simulink model "SFS"  (R2026a)
settings: Solver=ode23t  StopTime=pp.t_stop  AbsTol=1e-3
PreLoadFcn:
  | addpath(fileparts(which('SFS')));
  | pp = protectionParams();
InitFcn:
  | addpath(fileparts(which('SFS')));
  | pp = protectionParams();
undefined symbols (not defined in the file or in its folder): DiscIntNeverNeededParam
libraries: ee_lib x5, fl_lib x4, nesl_utility x4
settings Model: Creator=smred  LastModifiedBy=smred
settings DebuggingCC: SymbolicDimsDataTypeCodeGenerationDiagnostic=none
settings SimscapeCC: SimscapeLogDecimation=50.0

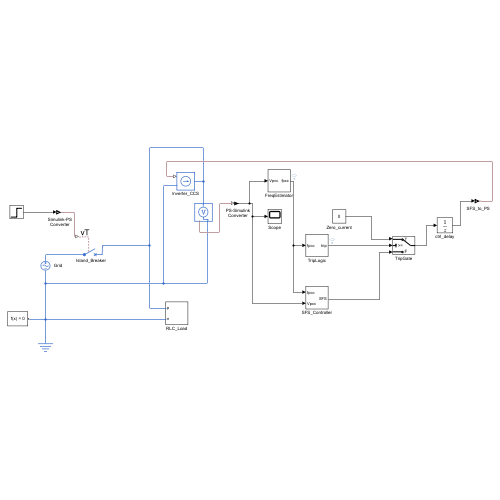
[thumbnail: Simulink's stored preview of the top-level diagram]
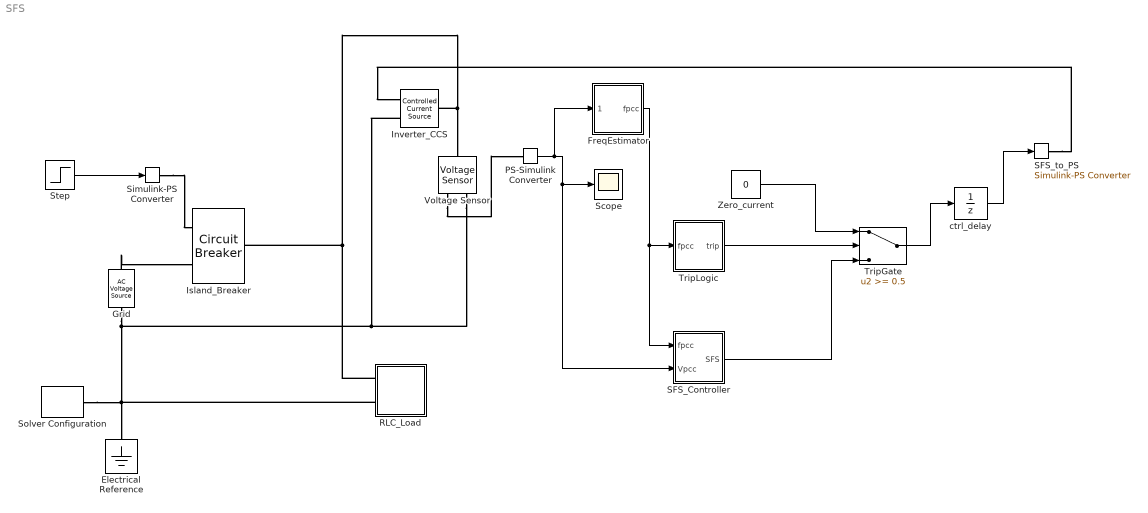
== system SFS ==
  Electrical Reference : fl_lib/Electrical/Electrical Elements/Electrical Reference
  FreqEstimator : Subsystem
  Grid : fl_lib/Electrical/Electrical Sources/AC Voltage Source  amp=pp.Vg_amp V  shift=0 deg  frequency=pp.f_n Hz
  Inverter_CCS : fl_lib/Electrical/Electrical Sources/Controlled Current Source
  Island_Breaker : ee_lib/Switches & Breakers/Circuit Breaker  R_closed=0.001 Ohm  G_open=1e-6 1/Ohm  threshold=0.5 V  breaker_behavior=ee.enum.switches.breakerBehavior.zeroCrossingDisable  port_option=ee.enum.threePhasePort.composite  control_port_option=ee.enum.controlport.ps  i_th=1e-8 A
  PS-Simulink Converter : nesl_utility/PS-Simulink Converter  PhysicalDomain=network_engine_domain  SubClassName=ps_output  LeftPortType=input  RightPortType=output  PseudoPeriodic=off  Frequencies=[]  VectorFormat=inherit  Unit=inherit  AffineConversion=off
  RLC_Load : Subsystem
  SFS_Controller : Subsystem
  SFS_to_PS : nesl_utility/Simulink-PS Converter  PhysicalDomain=network_engine_domain  SubClassName=ps_input  LeftPortType=input  RightPortType=output  PseudoPeriodic=off  Frequencies=[]  NoiseDistribution=none  NoiseParameters=[]  Unit=1  AffineConversion=off  FilteringAndDerivatives=zero  SimscapeFilterOrder=1  InputFilterTimeConstant=0.001  UdotUserProvided=0
  Scope : Scope
      settings: ActiveDisplayYMinimum=-408.578503188974  ActiveDisplayYMaximum=411.2206775988297
  Simulink-PS Converter : nesl_utility/Simulink-PS Converter  PhysicalDomain=network_engine_domain  SubClassName=ps_input  LeftPortType=input  RightPortType=output  PseudoPeriodic=off  Frequencies=[]  NoiseDistribution=none  NoiseParameters=[]  Unit=1  AffineConversion=off  FilteringAndDerivatives=provide  SimscapeFilterOrder=1  InputFilterTimeConstant=0.001  UdotUserProvided=0
  Solver Configuration : nesl_utility/Solver Configuration  PhysicalDomain=network_engine_domain  SubClassName=solver  LeftPortType=input  RightPortType=generic  Tones=[]  Harmonics=[]  SimulateNoise=off  Profile=off  UseLocalSampling=off  EnableSwitchedLinearOptims=on  FrequencyDomain=off  UseCCode=off  RelTol=0.001  AbsTol=0.001  MinStep=1e-09  ToWorkspace=off  RevertToSquareIcSolve=off  NumHomotopyIterations=100  PhasorMode=off  PhasorModeNumHarmonics=1  ConsistencySolver=NEWTON_XTOL_AFTER_FTOL  CanonicalOrdering=CANONICAL  OptimizeIntermediates=OPTIMIZED  IndexReductionMethod=DerivativeReplacement  DoDC=off  ResidualTolerance=1e-09  ConsistencyTolSource=GLOBAL  ConsistencyAbsTol=0.001  ConsistencyRelTol=0.001  ConsistencyTolFactor=0.001  UseLocalSolver=off  LocalSolverChoice=NE_BACKWARD_EULER_ADVANCER  ResolveIndetEquations=on  FunctionEvalNumThread=1  LocalSolverSampleTime=0.001  DoFixedCost=off  MaxNonlinIter=3  MaxModeIter=2  ComputeImpulses=off  ImpulseIterations=2  LinearAlgebra=auto  LinearAlgebraNumThread=0  EquationFormulation=NE_TIME_EF  DelaysMemoryBudget=1024  AutomaticFiltering=on  FilteringTimeConstant=0.001  PartitionStorageMethod=AS_NEEDED  PartitionMemoryBudget=1024  PartitionMethod=ROBUST  MultibodyUseLocalSolver=off  MultibodyLocalSolverChoice=ODE1  MultibodyLocalSolverSampleTime=0.001
  Step : Step  Time=pp.t_island  SampleTime=0
  TripGate : Switch  Threshold=0.5  SaturateOnIntegerOverflow=off  InputSameDT=off
  TripLogic : Subsystem
  Voltage Sensor : fl_lib/Electrical/Electrical Sensors/Voltage Sensor
  Zero_current : Constant  Value=0
  ctrl_delay : UnitDelay  SampleTime=pp.Ts
  wires:
  Step/1 -> Simulink-PS Converter/1
  ctrl_delay/1 -> SFS_to_PS/1
  FreqEstimator/1(fpcc) -> SFS_Controller/1(fpcc), TripLogic/1(fpcc)
  SFS_Controller/1(SFS) -> TripGate/3
  PS-Simulink Converter/1 -> Scope/1, SFS_Controller/2(Vpcc), FreqEstimator/1(Vpcc)
  Zero_current/1 -> TripGate/1
  TripLogic/1(trip) -> TripGate/2
  TripGate/1 -> ctrl_delay/1
  connections:
  Voltage Sensor/RConn2 -- Inverter_CCS/RConn2 -- Electrical Reference/LConn1 -- Solver Configuration/RConn1 -- RLC_Load/LConn2 -- Grid/RConn1
  Grid/LConn1 -- Island_Breaker/LConn2
  Simulink-PS Converter/RConn1 -- Island_Breaker/LConn1
  Island_Breaker/RConn1 -- Inverter_CCS/LConn1 -- Voltage Sensor/LConn1 -- RLC_Load/LConn1
  Voltage Sensor/RConn1 -- PS-Simulink Converter/LConn1
  SFS_to_PS/RConn1 -- Inverter_CCS/RConn1

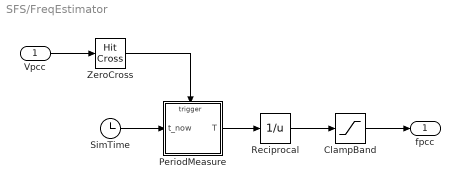
== system SFS/FreqEstimator ==
  Vpcc : Inport
  ClampBand : Saturate  UpperLimit=55  LowerLimit=45
  PeriodMeasure : Subsystem
  Reciprocal : Math  Operator=reciprocal
  SimTime : Clock
  ZeroCross : HitCross  HitCrossingDirection=rising
  fpcc : Outport
  wires:
  ClampBand/1 -> fpcc/1
  Reciprocal/1 -> ClampBand/1
  PeriodMeasure/1(T) -> Reciprocal/1
  ZeroCross/1 -> PeriodMeasure/Trigger
  SimTime/1 -> PeriodMeasure/1(t_now)
  Vpcc/1 -> ZeroCross/1

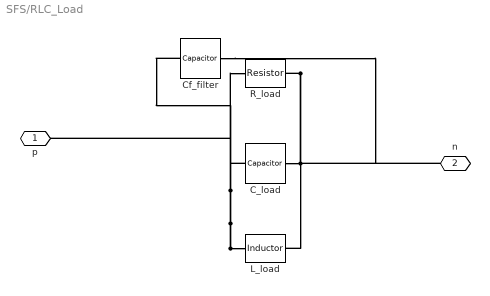
== system SFS/RLC_Load ==
  C_load : ee_lib/Passive/Capacitor  cap_option=ee.enum.passive.capacitor.capOption.const  c=pp.C_load F  Cvec=[1e-05, 1e-06] F  Vvec=[0, 10] V  CV_table_symmetry=ee.enum.passive.capacitor.tableSymmetry.yes  f_vec=[1, 10] kHz  DFext_vec=[.8, 1.2]  enable_C_tol=ee.enum.toleranceApplication.none  averaging_period=0 s  C_tol=5  tol_distribution=ee.enum.toleranceDistribution.uniform  nSigma=4  r=0 Ohm  g=0 1/Ohm  enable_operating_limits=ee.enum.enable.no  operating_limit_action=ee.enum.passive.reportOpLim.warn  max_working_voltage_range=[-25, 25] V  power_rating=1 W  maxTemperature=85 degC  thermalEnable=false  thermalMass=1 J/K  i_specify=off  i_priority=None  i=0 A  i_nominal_specify=off  i_nominal_value=1  i_nominal_unit=A  v_specify=off  v_priority=None  v=0 V  v_nominal_specify=off  v_nominal_value=1  v_nominal_unit=V  vc_specify=off  vc_priority=High  vc=0 V  vc_nominal_specify=off  vc_nominal_value=1  vc_nominal_unit=V  T_specify=off  T_priority=None  T=298.15 K  T_nominal_specify=off  T_nominal_value=1  T_nominal_unit=K
  Cf_filter : ee_lib/Passive/Capacitor  cap_option=ee.enum.passive.capacitor.capOption.const  c=pp.Cf F  Cvec=[1e-05, 1e-06] F  Vvec=[0, 10] V  CV_table_symmetry=ee.enum.passive.capacitor.tableSymmetry.yes  f_vec=[1, 10] kHz  DFext_vec=[.8, 1.2]  enable_C_tol=ee.enum.toleranceApplication.none  averaging_period=0 s  C_tol=5  tol_distribution=ee.enum.toleranceDistribution.uniform  nSigma=4  r=0 Ohm  g=0 1/Ohm  enable_operating_limits=ee.enum.enable.no  operating_limit_action=ee.enum.passive.reportOpLim.warn  max_working_voltage_range=[-25, 25] V  power_rating=1 W  maxTemperature=85 degC  thermalEnable=false  thermalMass=1 J/K  i_specify=off  i_priority=None  i=0 A  i_nominal_specify=off  i_nominal_value=1  i_nominal_unit=A  v_specify=off  v_priority=None  v=0 V  v_nominal_specify=off  v_nominal_value=1  v_nominal_unit=V  vc_specify=off  vc_priority=High  vc=0 V  vc_nominal_specify=off  vc_nominal_value=1  vc_nominal_unit=V  T_specify=off  T_priority=None  T=298.15 K  T_nominal_specify=off  T_nominal_value=1  T_nominal_unit=K
  L_load : ee_lib/Passive/Inductor  l=pp.L_load H  enable_L_tol=ee.enum.toleranceApplication.none  L_tol=20  tol_distribution=ee.enum.toleranceDistribution.uniform  nSigma=4  r=0 Ohm  g=1e-9 1/Ohm  enable_operating_limits=ee.enum.enable.no  operating_limit_action=ee.enum.passive.reportOpLim.warn  max_working_current=1 A  power_rating=1 W  i_L_specify=on  i_L_priority=High  i_L=pp.iL0 A  i_L_nominal_specify=off  i_L_nominal_value=1  i_L_nominal_unit=A
  R_load : ee_lib/Passive/Resistor  R=pp.R_load Ohm  enable_R_tol=ee.enum.toleranceApplication.none  R_tol=5  tol_distribution=ee.enum.toleranceDistribution.uniform  nSigma=4  enable_operating_limits=ee.enum.enable.no  operating_limit_action=ee.enum.passive.reportOpLim.warn  power_rating=1 W  max_working_voltage=100 V  noise_mode=ee.enum.sources.noise.Disabled  Tdevice=25 degC  sample_time=1e-3 s  repeatability=ee.enum.ic.repeatability.notRepeatable  user_seed=0  auto_seed=1045931777  power_derating_T1=70 degC  power_derating_T2=155 degC  operating_temperature_range_vec=[-50, 150] degC  alpha=3.93e-3 1/K  Tmeas=25 degC  thermal_mass=100 J/K  temperature_specify=off  temperature_priority=High  temperature=298.15 K  temperature_nominal_specify=off  temperature_nominal_value=1  temperature_nominal_unit=K
  p : PMIOPort  Side=Left
  n : PMIOPort  Port=2  Side=Left
  connections:
  L_load/LConn1 -- Cf_filter/LConn1 -- R_load/LConn1 -- p/RConn1 -- C_load/LConn1
  R_load/RConn1 -- n/RConn1 -- Cf_filter/RConn1 -- L_load/RConn1 -- C_load/RConn1

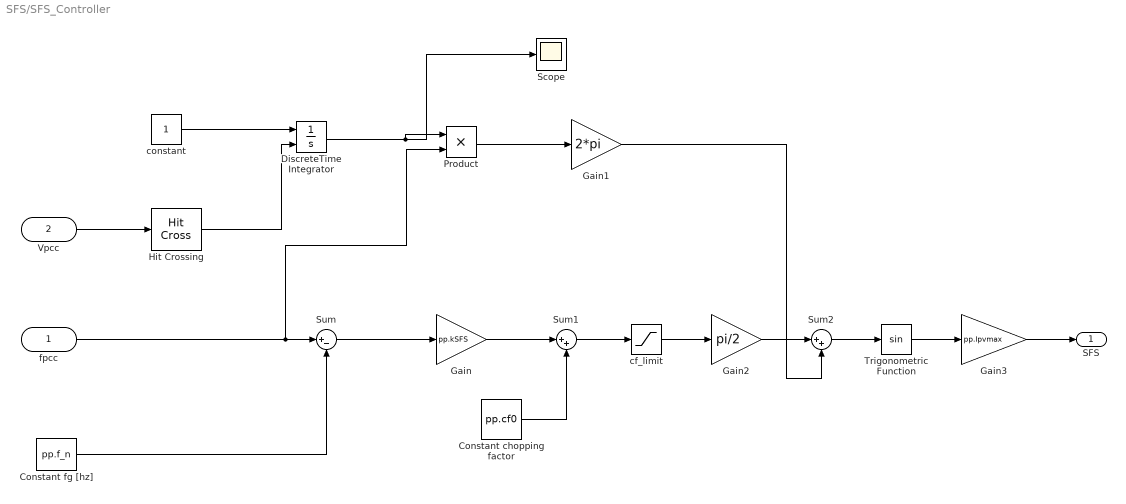
== system SFS/SFS_Controller ==
  fpcc : Inport
  Vpcc : Inport  Port=2
  Constant chopping factor : Constant  Value=pp.cf0
  Constant fg [hz] : Constant  Value=pp.f_n
  DiscreteTime Integrator : Integrator  ExternalReset=rising
  Gain : Gain  Gain=pp.kSFS
  Gain1 : Gain  Gain=2*pi
  Gain2 : Gain  Gain=pi/2
  Gain3 : Gain  Gain=pp.Ipvmax
  Hit Crossing : HitCross  HitCrossingDirection=rising  ZeroCross=off
  Product : Product
  Scope : Scope
      settings: ActiveDisplayYMinimum=-1  ActiveDisplayYMaximum=1
  Sum : Sum  Inputs=|+-
  Sum1 : Sum  Inputs=|++
  Sum2 : Sum  Inputs=|++
  Trigonometric Function : Trigonometry
  cf_limit : Saturate  UpperLimit=pp.cf_max  LowerLimit=-pp.cf_max
  constant : Constant
  SFS : Outport
  wires:
  Vpcc/1 -> Hit Crossing/1
  fpcc/1 -> Product/2, Sum/1
  Constant fg [hz]/1 -> Sum/2
  Sum/1 -> Gain/1
  Product/1 -> Gain1/1
  Gain/1 -> Sum1/1
  Constant chopping factor/1 -> Sum1/2
  constant/1 -> DiscreteTime Integrator/1
  Hit Crossing/1 -> DiscreteTime Integrator/2
  DiscreteTime Integrator/1 -> Scope/1, Product/1
  cf_limit/1 -> Gain2/1
  Gain3/1 -> SFS/1
  Trigonometric Function/1 -> Gain3/1
  Sum2/1 -> Trigonometric Function/1
  Gain1/1 -> Sum2/2
  Gain2/1 -> Sum2/1
  Sum1/1 -> cf_limit/1

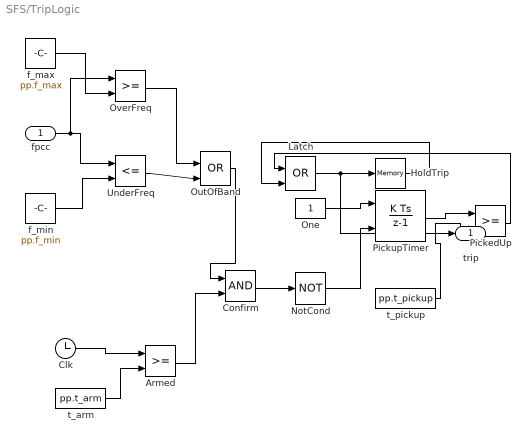
== system SFS/TripLogic ==
  fpcc : Inport
  Armed : RelationalOperator  OutDataTypeStr=boolean  RndMeth=Simplest  InputSameDT=off
  Clk : Clock
  Confirm : Logic  AllPortsSameDT=off  OutDataTypeStr=boolean
  HoldTrip : Memory
  Latch : Logic  Operator=OR  IconShape=distinctive  AllPortsSameDT=off  OutDataTypeStr=boolean
  NotCond : Logic  Operator=NOT  Inputs=1  AllPortsSameDT=off  OutDataTypeStr=boolean
  One : Constant
  OutOfBand : Logic  Operator=OR  IconShape=distinctive  AllPortsSameDT=off  OutDataTypeStr=boolean
  OverFreq : RelationalOperator  OutDataTypeStr=boolean  RndMeth=Simplest  InputSameDT=off
  PickedUp : RelationalOperator  OutDataTypeStr=boolean  RndMeth=Simplest  InputSameDT=off
  PickupTimer : DiscreteIntegrator  gainval=1  ExternalReset=level  SampleTime=pp.Ts  ICPrevOutput=DiscIntNeverNeededParam  ICPrevScaledInput=DiscIntNeverNeededParam
  UnderFreq : RelationalOperator  Operator=<=  OutDataTypeStr=boolean  RndMeth=Simplest  InputSameDT=off
  f_max : Constant  Value=pp.f_max
  f_min : Constant  Value=pp.f_min
  t_arm : Constant  Value=pp.t_arm
  t_pickup : Constant  Value=pp.t_pickup
  trip : Outport
  wires:
  fpcc/1 -> UnderFreq/1, OverFreq/1
  f_max/1 -> OverFreq/2
  f_min/1 -> UnderFreq/2
  OverFreq/1 -> OutOfBand/1
  UnderFreq/1 -> OutOfBand/2
  HoldTrip/1 -> Latch/2
  Latch/1 -> trip/1, HoldTrip/1
  Clk/1 -> Armed/1
  t_arm/1 -> Armed/2
  OutOfBand/1 -> Confirm/1
  Armed/1 -> Confirm/2
  Confirm/1 -> NotCond/1
  One/1 -> PickupTimer/1
  NotCond/1 -> PickupTimer/2
  PickupTimer/1 -> PickedUp/1
  t_pickup/1 -> PickedUp/2
  PickedUp/1 -> Latch/1

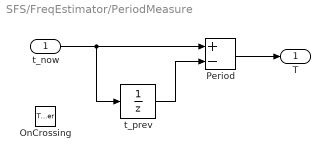
== system SFS/FreqEstimator/PeriodMeasure ==
  t_now : Inport
  OnCrossing : TriggerPort  VariantControl=(inherit)  PortDimensions=1
  Period : Sum  Inputs=+-
  t_prev : UnitDelay  InitialCondition=-1/pp.f_n  SampleTime=-1
  T : Outport  InitialOutput=1/pp.f_n
  wires:
  Period/1 -> T/1
  t_prev/1 -> Period/2
  t_now/1 -> t_prev/1, Period/1
